simulink model "EjEcualizador"  (Simulink 8.6)
settings: Solver=ode45  StartTime=0.0  StopTime=inf  RelTol=1e-3
libraries: powerlib x10, dspvision x1, dspsnks4 x1
settings Model: Creator=Milton  LastModifiedBy=fernando
settings DebuggingCC: FcnCallInpInsideContextMsg=UseLocalSettings

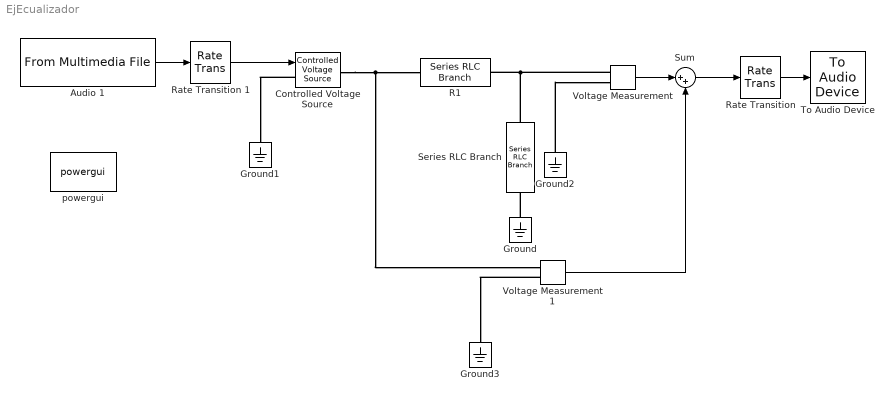
== system EjEcualizador ==
  Audio 1 : dspvision/From Multimedia File  inputFilename=mono_the_3_tenors_o_sole_mio_994_converted.wav  loop=on  numPlays=inf  outputStreams=Audio only  videoDataType=single  audioDataType=double  inheritSampleTime=on  userDefinedSampleTime=1/30  noAudioOutput=off  isIntensityVideo=off  fourcc=RGB  colorVideoFormat=Separate color signals  outputEOF=off  dataOrg=Column-major  audioFrameSize=1  computeAudioFrameSize=off  outSamplingMode=Frame based
  Controlled Voltage Source : powerlib/Electrical Sources/Controlled Voltage Source  Initialize=on  Source_Type=AC  Amplitude=0  Phase=0  Frequency=0  Measurements=None
  Ground{,1..3} (4 alike) : powerlib/Elements/Ground  LConnTagsString=a
  R1 : powerlib/Elements/Series RLC Branch  LConnTagsString=__new0  RConnTagsString=__new0  BranchType=R  Resistance=1000*(1/(2*pi))  Inductance=1e-3  SetiL0=off  InitialCurrent=0  Capacitance=1e-6  Setx0=off  InitialVoltage=0  Measurements=None
  Rate Transition : RateTransition  OutPortSampleTime=1/8000
  Rate Transition 1 : RateTransition
  Series RLC Branch : powerlib/Elements/Series RLC Branch  LConnTagsString=__new0  RConnTagsString=__new0  BranchType=C  Resistance=1  Inductance=1e-3  SetiL0=off  InitialCurrent=0  Capacitance=0.000001  Setx0=off  InitialVoltage=0  Measurements=None
  Sum : Sum  Inputs=|++
  To Audio Device : dspsnks4/To Audio Device  deviceName=Default  inheritSampleRate=off  sampleRate=8000  deviceDatatype=Determine from input data type  autoBufferSize=on  bufferSize=4096  queueDuration=1.0  defaultOutputChannelMapping=on  outputChannelMapping=1:2  outputNumUnderrunSamples=off
  Voltage Measurement : powerlib/Measurements/Voltage Measurement  PhasorSimulation=off  OutputType=Complex  PSBequivalent=0
  Voltage Measurement1 : powerlib/Measurements/Voltage Measurement  PhasorSimulation=off  OutputType=Complex  PSBequivalent=0
  powergui : powerlib/powergui  Priority=1  SimulationMode=Continuous  SolverType=Tustin  SampleTime=50e-6  frequency=60  SPID=off  DisableSnubberDevices=off  DisableRonSwitches=off  DisableVfSwitches=off  SwTol=0  DisplayEquations=off  Interpol=off  ExternalGateDelay=off  methode=off  Ts=10  FunctionMessages=off  echomessages=off  HookPort=off  EnableUseOfTLC=off  x0status=blocks  frequencyindice=0  Pbase=100e6  ErrMax=1e-4  Iterations=50  UnitsV=kV  UnitsW=MW  buscounter=0  RestoreLinks=warning  ResistiveCurrentMeasurement=off  Frange=[0:2:500]  Ylog=off  Xlog=on  ShowGrid=off  save=off  variable=ZData  structure=0  ZoomFFT=off  StartTime=0.0  cycles=1  DisplayStyle=1  fundamental=60  FreqAxis=off  MaxFrequency=1000  frequencyindicesteady=1  RmsSteady=1  display=off
  wires:
  Audio 1/1 -> Rate Transition 1/1
  Rate Transition/1 -> To Audio Device/1
  Rate Transition 1/1 -> Controlled Voltage Source/1
  Sum/1 -> Rate Transition/1
  Voltage Measurement/1 -> Sum/1
  Voltage Measurement1/1 -> Sum/2
  connections:
  Controlled Voltage Source/RConn1 -- R1/LConn1 -- Voltage Measurement1/LConn1
  Ground/LConn1 -- Series RLC Branch/RConn1
  Controlled Voltage Source/LConn1 -- Ground1/LConn1
  Ground2/LConn1 -- Voltage Measurement/LConn2
  Voltage Measurement1/LConn2 -- Ground3/LConn1
  Voltage Measurement/LConn1 -- Series RLC Branch/LConn1 -- R1/RConn1
